simulink model "FMstereo"  (Simulink 10.1)
settings: Solver=FixedStepDiscrete  StartTime=0.0  StopTime=inf  RelTol=1e-3
PreLoadFcn:
  | setenv('MW_MINGW64_LOC','C:\TDM-GCC-64')
StartFcn:
  | tic
StopFcn:
  | toc;
undefined symbols (not defined in the file): magnitude
libraries: dsparch4 x5, UN_HIL_Lib x4, dspobslib x3, dspswit3 x1, commsynccomp2 x1
Description:
  | QPSK Transmitter and Receiver.
  | 
  | This model shows the implementation of a QPSK transmitter and receiver.
settings Model: FPTRunName=Active  Creator=The MathWorks Inc.  LastModifiedBy=THINKPAD
settings DataIOCC: LimitDataPoints=on  SignalLoggingSaveFormat=ModelDataLogs  SaveOutput=off  SaveTime=off
settings OptimizationCC: BooleanDataType=off  DefaultParameterBehavior=Inlined  ExpressionDepthLimit=2147483647  LocalBlockOutputs=off
settings DebuggingCC: AlgebraicLoopMsg=error  SolverPrmCheckMsg=warning  SingleTaskRateTransMsg=error  ParameterPrecisionLossMsg=none  FcnCallInpInsideContextMsg=warning  StateNameClashWarn=warning
settings HardwareCC: TargetBitPerPointer=64  TargetBitPerSizeT=64  TargetBitPerPtrDiffT=64  TargetLongLongMode=on  TargetIntDivRoundTo=Zero  TargetEndianess=LittleEndian  TargetWordSize=64  TargetHWDeviceType=Generic->MATLAB Host Computer  ProdEqTarget=off
settings GRTTargetCC: CombineOutputUpdateFcns=on  GRTInterface=off
settings ConfigComp: CovSFcnEnable=off
settings SimEventsCC: propDiagStatOutput=1  propPreventDuplicateEvents=0

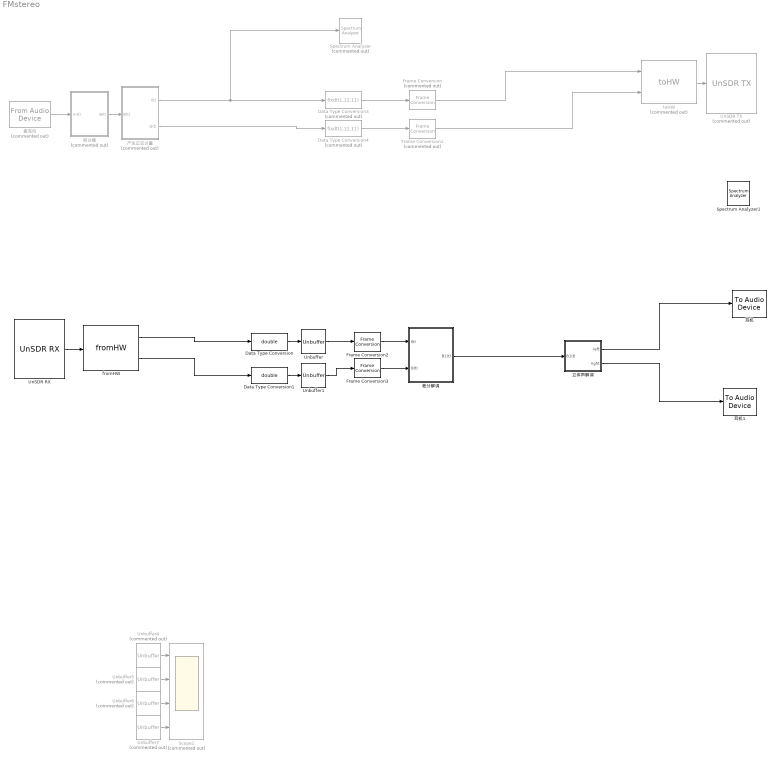
== system FMstereo ==
  Data Type Conversion : DataTypeConversion  OutDataTypeStr=double
  Data Type Conversion1 : DataTypeConversion  OutDataTypeStr=double
  Data Type Conversion3 : DataTypeConversion  Commented=on  OutDataTypeStr=fixdt(1,12,11)
  Data Type Conversion4 : DataTypeConversion  Commented=on  OutDataTypeStr=fixdt(1,12,11)
  Frame Conversion : FrameConversion  Commented=on  OutFrame=Sample-based
  Frame Conversion1 : FrameConversion  Commented=on  OutFrame=Sample-based
  Frame Conversion2 : FrameConversion  OutFrame=Sample-based
  Frame Conversion3 : FrameConversion  OutFrame=Sample-based
  Scope1 : Scope  Commented=on  NumInputPorts=4
  Spectrum Analyzer : SpectrumAnalyzer  Commented=on
  Spectrum Analyzer1 : SpectrumAnalyzer
  UnSDR RX : UN_HIL_Lib/UnSDR RX  SystemSampleTime=-1  Latency=0  AutoFrameSizeCalculation=off
      settings: SourceProductName=HIL Blockset
  UnSDR TX : UN_HIL_Lib/UnSDR TX  Commented=on  SystemSampleTime=-1  Latency=0  AutoFrameSizeCalculation=off
      settings: SourceProductName=HIL Blockset
  Unbuffer : Unbuffer
  Unbuffer1 : Unbuffer
  Unbuffer{4..7} (4 alike) : Unbuffer  Commented=on
  fromHW : UN_HIL_Lib/fromHW  sp=1/128e3
      settings: SourceProductName=HIL Blockset
  toHW : UN_HIL_Lib/toHW  Commented=on  SystemSampleTime=-1  Latency=0  AutoFrameSizeCalculation=off
      settings: SourceProductName=HIL Blockset
  产生正交分量 : Subsystem  Commented=on
  差分解调 : Subsystem
  积分器 : Subsystem  Commented=on
  立体声解调 : Subsystem
  耳机 : dspobslib/To Audio Device  deviceName=Default  inheritSampleRate=on  sampleRate=44100  deviceDatatype=Determine from input data type  autoBufferSize=on  bufferSize=4096  queueDuration=2  defaultOutputChannelMapping=on  outputChannelMapping=1:2  outputNumUnderrunSamples=off
      settings: SourceProductBaseCode=DS
  耳机1 : dspobslib/To Audio Device  deviceName=Default  inheritSampleRate=on  sampleRate=44100  deviceDatatype=Determine from input data type  autoBufferSize=on  bufferSize=4096  queueDuration=2  defaultOutputChannelMapping=on  outputChannelMapping=1:2  outputNumUnderrunSamples=off
      settings: SourceProductBaseCode=DS
  麦克风 : dspobslib/From Audio Device  Commented=on  deviceName=Default  numChannels=1  sampleRate=128000  deviceDatatype=Determine from output data type  autoBufferSize=on  bufferSize=4096  queueDuration=1.0  frameSize=1  outputDatatype=single  defaultInputChannelMapping=on  inputChannelMapping=1:2  outputNumOverrunSamples=off  OutputFrames=on
      settings: SourceProductBaseCode=DS
  wires:
  Unbuffer5/1 -> Scope1/2
  Unbuffer6/1 -> Scope1/3
  Unbuffer7/1 -> Scope1/4
  Unbuffer4/1 -> Scope1/1
  Data Type Conversion3/1 -> Frame Conversion/1
  Data Type Conversion4/1 -> Frame Conversion1/1
  Unbuffer/1 -> Frame Conversion2/1
  Data Type Conversion/1 -> Unbuffer/1
  麦克风/1 -> 积分器/1(m(t))
  积分器/1(B(t)) -> 产生正交分量/1(B(t))
  Data Type Conversion1/1 -> Unbuffer1/1
  Unbuffer1/1 -> Frame Conversion3/1
  产生正交分量/1(I(t)) -> Data Type Conversion3/1, Spectrum Analyzer/1
  产生正交分量/2(Q(t)) -> Data Type Conversion4/1
  Frame Conversion2/1 -> 差分解调/1(I(t))
  Frame Conversion3/1 -> 差分解调/2(Q(t))
  toHW/1 -> UnSDR TX/1
  UnSDR RX/1 -> fromHW/1
  fromHW/1 -> Data Type Conversion/1
  fromHW/2 -> Data Type Conversion1/1
  Frame Conversion/1 -> toHW/1
  Frame Conversion1/1 -> toHW/2
  差分解调/1(B1(t)) -> 立体声解调/1(B1(t))
  立体声解调/1(left) -> 耳机/1
  立体声解调/2(right) -> 耳机1/1
  ? -> Spectrum Analyzer1/1

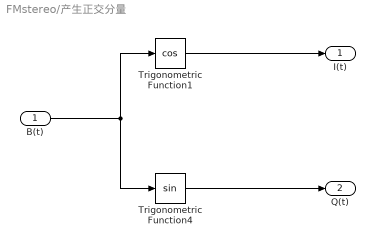
== system FMstereo/产生正交分量 ==
  B(t) : Inport
  Trigonometric Function1 : Trigonometry  Operator=cos  NumberOfIterations=16
  Trigonometric Function4 : Trigonometry  NumberOfIterations=16
  I(t) : Outport  VectorParamsAs1DForOutWhenUnconnected=off
  Q(t) : Outport  Port=2  VectorParamsAs1DForOutWhenUnconnected=off
  wires:
  Trigonometric Function1/1 -> I(t)/1
  B(t)/1 -> Trigonometric Function4/1, Trigonometric Function1/1
  Trigonometric Function4/1 -> Q(t)/1

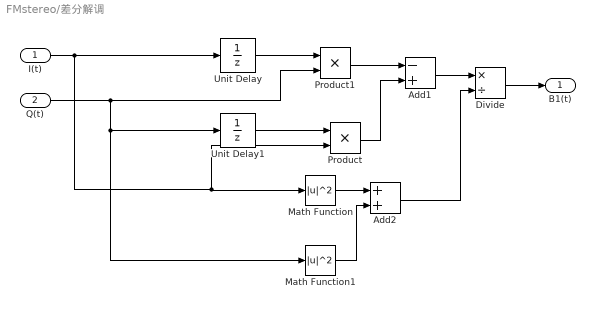
== system FMstereo/差分解调 ==
  I(t) : Inport
  Q(t) : Inport  Port=2
  Add1 : Sum  Inputs=-+
  Add2 : Sum
  Divide : Product  Inputs=*/
  Math Function : Math  Operator=magnitude^2  SignedPower=on  SaturateOnIntegerOverflow=on
  Math Function1 : Math  Operator=magnitude^2  SignedPower=on  SaturateOnIntegerOverflow=on
  Product : Product  RndMeth=Zero
  Product1 : Product  RndMeth=Zero
  Unit Delay : UnitDelay  SampleTime=-1  HasFrameUpgradeWarning=on
  Unit Delay1 : UnitDelay  SampleTime=-1  HasFrameUpgradeWarning=on
  B1(t) : Outport  VectorParamsAs1DForOutWhenUnconnected=off
  wires:
  Add1/1 -> Divide/1
  Add2/1 -> Divide/2
  Product/1 -> Add1/2
  Product1/1 -> Add1/1
  Unit Delay/1 -> Product1/1
  Unit Delay1/1 -> Product/1
  Q(t)/1 -> Math Function1/1, Unit Delay1/1, Product1/2
  I(t)/1 -> Product/2, Math Function/1, Unit Delay/1
  Math Function/1 -> Add2/1
  Math Function1/1 -> Add2/2
  Divide/1 -> B1(t)/1

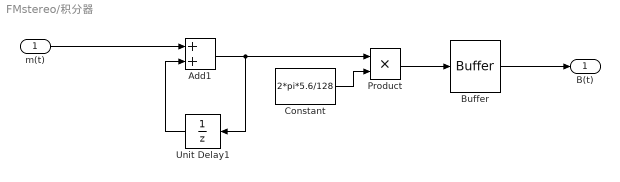
== system FMstereo/积分器 ==
  m(t) : Inport
  Add1 : Sum  OutDataTypeStr=Inherit: Same as first input
  Buffer : Buffer  N=4096
  Constant : Constant  Value=2*pi*5.6/128  VectorParams1D=off  SampleTime=-1
  Product : Product  RndMeth=Zero  OutDataTypeStr=Inherit: Same as first input
  Unit Delay1 : UnitDelay  SampleTime=-1  HasFrameUpgradeWarning=on
  B(t) : Outport  VectorParamsAs1DForOutWhenUnconnected=off
  wires:
  Product/1 -> Buffer/1
  Constant/1 -> Product/2
  Add1/1 -> Product/1, Unit Delay1/1
  Unit Delay1/1 -> Add1/2
  m(t)/1 -> Add1/1
  Buffer/1 -> B(t)/1

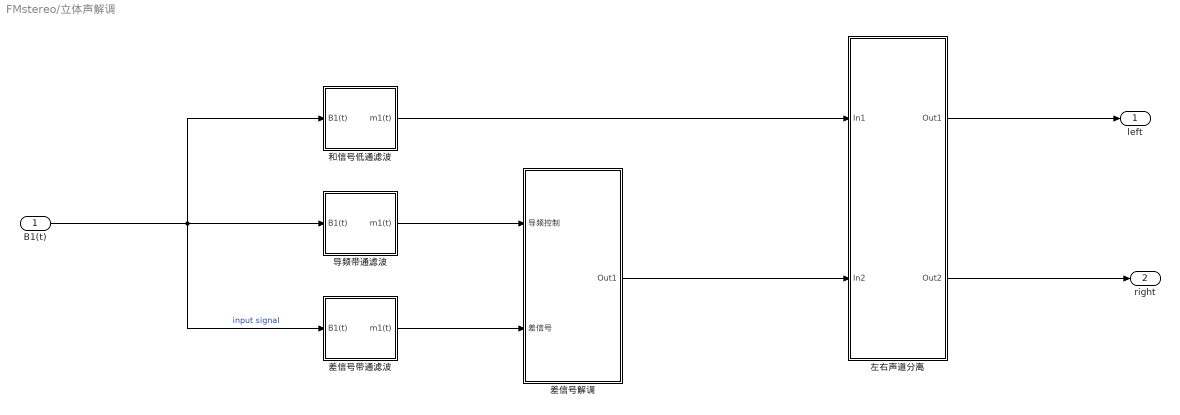
== system FMstereo/立体声解调 ==
  B1(t) : Inport
  和信号低通滤波 : Subsystem
  导频带通滤波 : Subsystem
  左右声道分离 : Subsystem
  差信号带通滤波 : Subsystem
  差信号解调 : Subsystem
  left : Outport
  right : Outport  Port=2
  wires:
  B1(t)/1 -> 差信号带通滤波/1(B1(t)), 导频带通滤波/1(B1(t)), 和信号低通滤波/1(B1(t))  "input signal"
  导频带通滤波/1(m1(t)) -> 差信号解调/1(导频控制)
  差信号带通滤波/1(m1(t)) -> 差信号解调/2(差信号)
  和信号低通滤波/1(m1(t)) -> 左右声道分离/1(In1)
  差信号解调/1(Out1) -> 左右声道分离/2(In2)
  左右声道分离/1(Out1) -> left/1
  左右声道分离/2(Out2) -> right/1

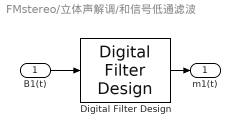
== system FMstereo/立体声解调/和信号低通滤波 ==
  B1(t) : Inport
  Digital Filter Design : dsparch4/Digital Filter Design  mwdsp_browser_bugfix_var=off
  m1(t) : Outport  VectorParamsAs1DForOutWhenUnconnected=off
  wires:
  B1(t)/1 -> Digital Filter Design/1
  Digital Filter Design/1 -> m1(t)/1

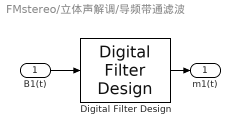
== system FMstereo/立体声解调/导频带通滤波 ==
  B1(t) : Inport
  Digital Filter Design : dsparch4/Digital Filter Design  mwdsp_browser_bugfix_var=off
  m1(t) : Outport  VectorParamsAs1DForOutWhenUnconnected=off
  wires:
  B1(t)/1 -> Digital Filter Design/1
  Digital Filter Design/1 -> m1(t)/1

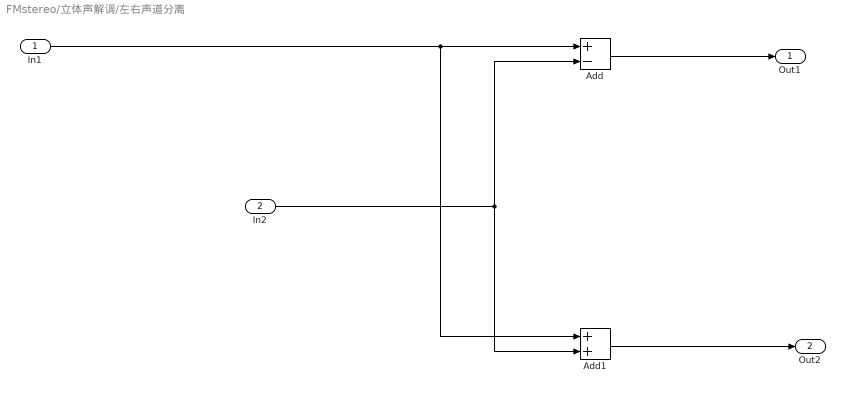
== system FMstereo/立体声解调/左右声道分离 ==
  In1 : Inport
  In2 : Inport  Port=2
  Add : Sum  Inputs=+-
  Add1 : Sum
  Out1 : Outport
  Out2 : Outport  Port=2
  wires:
  In1/1 -> Add1/1, Add/1
  In2/1 -> Add1/2, Add/2
  Add1/1 -> Out2/1
  Add/1 -> Out1/1

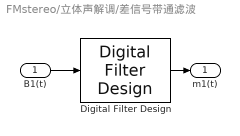
== system FMstereo/立体声解调/差信号带通滤波 ==
  B1(t) : Inport
  Digital Filter Design : dsparch4/Digital Filter Design  mwdsp_browser_bugfix_var=off
  m1(t) : Outport  VectorParamsAs1DForOutWhenUnconnected=off
  wires:
  B1(t)/1 -> Digital Filter Design/1
  Digital Filter Design/1 -> m1(t)/1

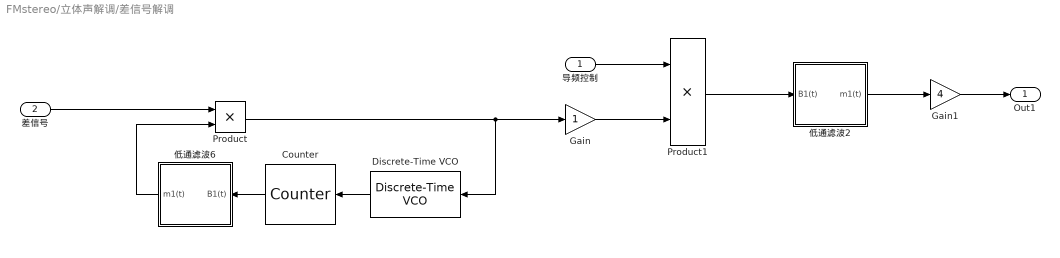
== system FMstereo/立体声解调/差信号解调 ==
  导频控制 : Inport
  差信号 : Inport  Port=2
  Counter : dspswit3/Counter  Direction=Up  CountEvent=Rising edge  CounterSize=8 bits  MaxCount=255  InitialCount=0  Output=Count  HitValue=32  ResetInput=off  SamplesPerFrame=1  Ts=1  CntDtype=double  HitDtype=Logical
  Discrete-Time VCO : commsynccomp2/Discrete-Time VCO  Ac=1  Fc=10  Kc=1  Ph=0  ts=0.01
      settings: SourceProductBaseCode=CM
  Gain : Gain
  Gain1 : Gain  Gain=4
  Product : Product
  Product1 : Product
  低通滤波2 : Subsystem
  低通滤波6 : Subsystem
  Out1 : Outport
  wires:
  Product1/1 -> 低通滤波2/1(B1(t))
  Product/1 -> Discrete-Time VCO/1, Gain/1
  导频控制/1 -> Product1/1
  Counter/1 -> 低通滤波6/1(B1(t))
  差信号/1 -> Product/1
  Gain/1 -> Product1/2
  Discrete-Time VCO/1 -> Counter/1
  低通滤波6/1(m1(t)) -> Product/2
  低通滤波2/1(m1(t)) -> Gain1/1
  Gain1/1 -> Out1/1

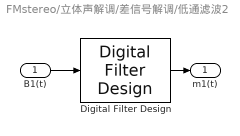
== system FMstereo/立体声解调/差信号解调/低通滤波2 ==
  B1(t) : Inport
  Digital Filter Design : dsparch4/Digital Filter Design  mwdsp_browser_bugfix_var=off
  m1(t) : Outport  VectorParamsAs1DForOutWhenUnconnected=off
  wires:
  B1(t)/1 -> Digital Filter Design/1
  Digital Filter Design/1 -> m1(t)/1

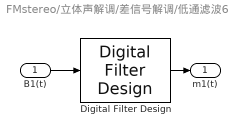
== system FMstereo/立体声解调/差信号解调/低通滤波6 ==
  B1(t) : Inport
  Digital Filter Design : dsparch4/Digital Filter Design  mwdsp_browser_bugfix_var=off
  m1(t) : Outport  VectorParamsAs1DForOutWhenUnconnected=off
  wires:
  B1(t)/1 -> Digital Filter Design/1
  Digital Filter Design/1 -> m1(t)/1
